simulink model "GSAutopilot"  (R2022b)
settings: Solver=ode45  StartTime=0.0  StopTime=50  RelTol=1e-3  AbsTol=1e-6
PreLoadFcn:
  | x_ini = 0;
  | h_ini = 10000/3.28084;  % 10,000 ft
  | alpha_ini = 0;
  | theta_ini = 0;
  | v_ini = 700;   % m/s
  | q_ini = 0;
model workspace (MATLAB code in the model file):
  | AirframeData
  | Kp0 = 0.1*ones(11,8);
  | Ki0 = 2*ones(11,8);
  | Ka0 = 0.001*ones(11,8);
  | Kg0 = -1000*ones(11,8);
values from neighbouring files (symbols this model uses):
  Cm_alpha = am*al.^3 + bm*al.*abs(al) - cm*(7-8*M/3).*al    [AirframeData.m]
  Cm_el = -0.206000/d2r    (= -11.8029305797)    [AirframeData.m]
  Cm_q = -1.719    [AirframeData.m]
  Cx_alpha = -0.3*ones(length(alpha_vec),length(Mach_vec))    [AirframeData.m]
  Cz_alpha = an*al.^3 + bn*al.*abs(al) + cn*(2-M/3).*al    [AirframeData.m]
  Cz_el = -0.034000/d2r    (= -1.94805650344)    [AirframeData.m]
  d2r = pi/180    (= 0.0174532925199)    [AirframeData.m]
  d_ref = 0.75/m2ft    (= 0.228599992685)    [AirframeData.m]
  fin_max = 30.0*d2r    (= 0.523598775598)    [AirframeData.m]
  fin_min = -30.0*d2r    (= -0.523598775598)    [AirframeData.m]
  g = 9.81    [AirframeData.m]
  S_ref = 0.44/m2ft^2    (= 0.0408773349839)    [AirframeData.m]
  Thrust = 10e3    (= 10000)    [AirframeData.m]
libraries: aerospace x2, simulink x1
settings Model: Creator=The MathWorks, Inc.  LastModifiedBy=cosorio
settings SolverCC: AutoScaleAbsTol=off  AlgebraicLoopSolver=TrustRegion
settings DataIOCC: SaveFormat=Array  ReturnWorkspaceOutputs=off  SignalLoggingName=sigsOut
settings OptimizationCC: BlockReduction=off  BooleanDataType=off  ExpressionDepthLimit=2147483647  InitFltsAndDblsToZero=on  LifeSpan=inf
settings DebuggingCC: SaveWithParameterizedLinksMsg=none  UnderspecifiedInitializationDetection=Classic  MergeDetectMultiDrivingBlocksExec=none  CheckExecutionContextPreStartOutputMsg=on  SignalResolutionControl=TryResolveAllWithWarning  MultiTaskDSMMsg=warning  FcnCallInpInsideContextMsg=warning  UnconnectedInputMsg=warning  UnconnectedOutputMsg=warning  UnconnectedLineMsg=warning  AllowSymbolicDim=off  StateNameClashWarn=warning  SFUnexpectedBacktrackingDiag=warning  SFNoUnconditionalDefaultTransitionDiag=warning  SFExecutionAtInitializationDiag=none  SFMachineParentedDataDiag=warning  ArithmeticOperatorsInVariantConditions=warning
settings HardwareCC: ProdBitPerPointer=32  ProdBitPerSizeT=32  ProdBitPerPtrDiffT=32  ProdLargestAtomicFloat=None  ProdIntDivRoundTo=Undefined  ProdEndianess=Unspecified  ProdWordSize=32  ProdHWDeviceType=32-bit Generic  TargetUnknown=on
settings ModelReferenceCC: EnableRefExpFcnMdlSchedulingChecks=on  PropagateSignalLabelsOutOfModel=off
settings SFSimCC: SimUseLocalCustomCode=off  CustomCodeUndefinedFunction=UseInterfaceOnly
settings RTWCC: RTWUseLocalCustomCode=off
settings CodeAppCC: StateflowObjectComments=on
settings GRTTargetCC: TargetFcnLib=ansi_tfl_tmw.mat  TargetLangStandard=C89/C90 (ANSI)  CombineOutputUpdateFcns=off  GRTInterface=on
settings ConfigComp: CovMetricSettings=dw  CovSaveCumulativeToWorkspaceVar=on  CovSaveSingleToWorkspaceVar=on  CovExternalEMLEnable=off

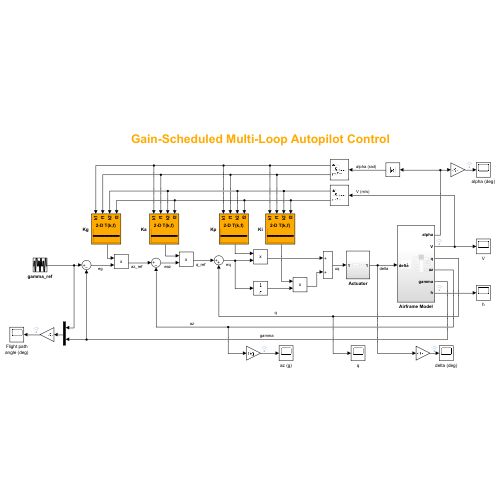
[thumbnail: Simulink's stored preview of the top-level diagram]
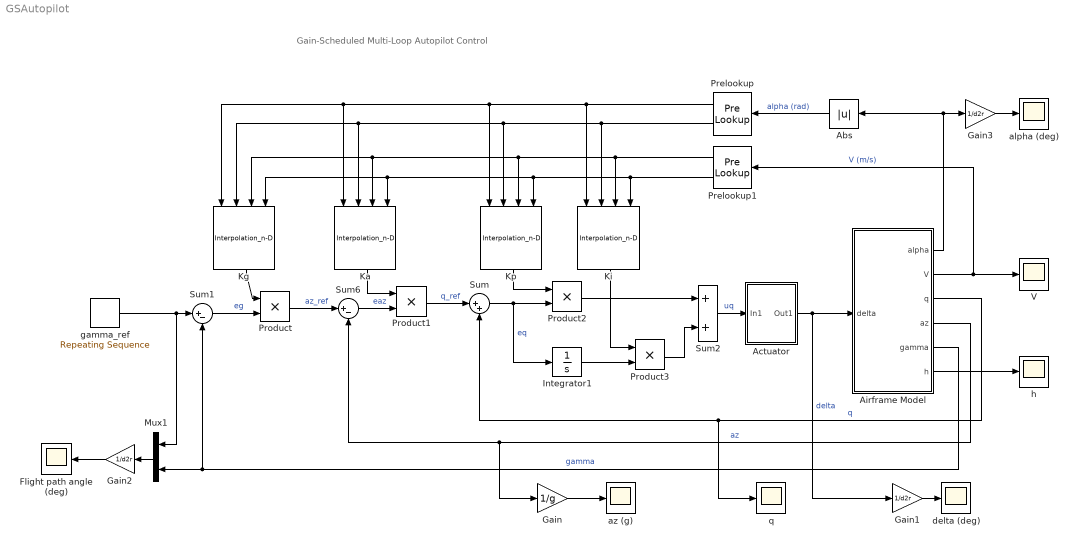
== system GSAutopilot ==
  note: Gain-Scheduled Multi-Loop Autopilot Control
  Abs : Abs  SaturateOnIntegerOverflow=off
  Actuator : Subsystem
  Airframe Model : Subsystem
  Flight path angle (deg) : Scope
  Gain : Gain  Gain=1/g
  Gain1 : Gain  Gain=1/d2r
  Gain2 : Gain  Gain=1/d2r
  Gain3 : Gain  Gain=1/d2r
  Integrator1 : Integrator
  Ka : Interpolation_n-D  Table=Ka0  InternalRulePriority=Speed
  Kg : Interpolation_n-D  Table=Kg0  InternalRulePriority=Speed
  Ki : Interpolation_n-D  Table=Ki0  InternalRulePriority=Speed
  Kp : Interpolation_n-D  Table=Kp0  InternalRulePriority=Speed
  Mux1 : Mux  Inputs=2
  Prelookup : PreLookup  BreakpointsData=(0:2:20)*(pi/180)  ExtrapMethod=Linear
  Prelookup1 : PreLookup  BreakpointsData=700:100:1400  ExtrapMethod=Linear
  Product{,1..3} (4 alike) : Product
  Sum : Sum  Inputs=|++  SaturateOnIntegerOverflow=on
  Sum1 : Sum  Inputs=|+-  SaturateOnIntegerOverflow=on
  Sum2 : Sum  SaturateOnIntegerOverflow=on
  Sum6 : Sum  Inputs=|+-  SaturateOnIntegerOverflow=on
  V : Scope
  alpha (deg) : Scope
  az (g) : Scope
  delta (deg) : Scope
  gamma_ref : simulink/Sources/Repeating Sequence  rep_seq_t=[0 6 8 16 20 26 32 40 44 50]  rep_seq_y=[0 0 pi/6 pi/6 -pi/6 -pi/6 pi/4 pi/4 0 0]
  h : Scope
  q : Scope
  wires:
  Sum/1 -> Product2/2, Integrator1/1  "eq"
  Product3/1 -> Sum2/2
  Airframe Model/4(az) -> Gain/1, Sum6/2  "az"
  Airframe Model/1(alpha) -> Abs/1, Gain3/1
  Product2/1 -> Sum2/1
  Product1/1 -> Sum/1  "q_ref"
  Sum6/1 -> Product1/2  "eaz"
  Actuator/1(Out1) -> Airframe Model/1(delta), Gain1/1  "delta"
  Product/1 -> Sum6/1  "az_ref"
  Sum1/1 -> Product/2  "eg"
  Airframe Model/5(gamma) -> Mux1/2, Sum1/2  "gamma"
  Sum2/1 -> Actuator/1(In1)  "uq"
  Airframe Model/3(q) -> q/1, Sum/2  "q"
  gamma_ref/1 -> Sum1/1, Mux1/1
  Gain/1 -> az (g)/1
  Gain1/1 -> delta (deg)/1
  Mux1/1 -> Gain2/1
  Gain2/1 -> Flight path angle (deg)/1
  Gain3/1 -> alpha (deg)/1
  Airframe Model/2(V) -> Prelookup1/1, V/1  "V (m/s)"
  Airframe Model/6(h) -> h/1
  Kg/1 -> Product/1
  Ka/1 -> Product1/1
  Integrator1/1 -> Product3/2
  Kp/1 -> Product2/1
  Ki/1 -> Product3/1
  Abs/1 -> Prelookup/1  "alpha (rad)"
  Prelookup/1 -> Ka/1, Kg/1, Kp/1, Ki/1
  Prelookup/2 -> Ki/2, Kp/2, Ka/2, Kg/2
  Prelookup1/1 -> Kp/3, Kg/3, Ka/3, Ki/3
  Prelookup1/2 -> Ki/4, Kg/4, Ka/4, Kp/4

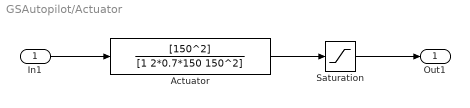
== system GSAutopilot/Actuator ==
  In1 : Inport
  Actuator : TransferFcn  Numerator=[150^2]  Denominator=[1 2*0.7*150 150^2]
  Saturation : Saturate  UpperLimit=fin_max  LowerLimit=fin_min
  Out1 : Outport  VectorParamsAs1DForOutWhenUnconnected=off
  wires:
  Actuator/1 -> Saturation/1
  In1/1 -> Actuator/1
  Saturation/1 -> Out1/1

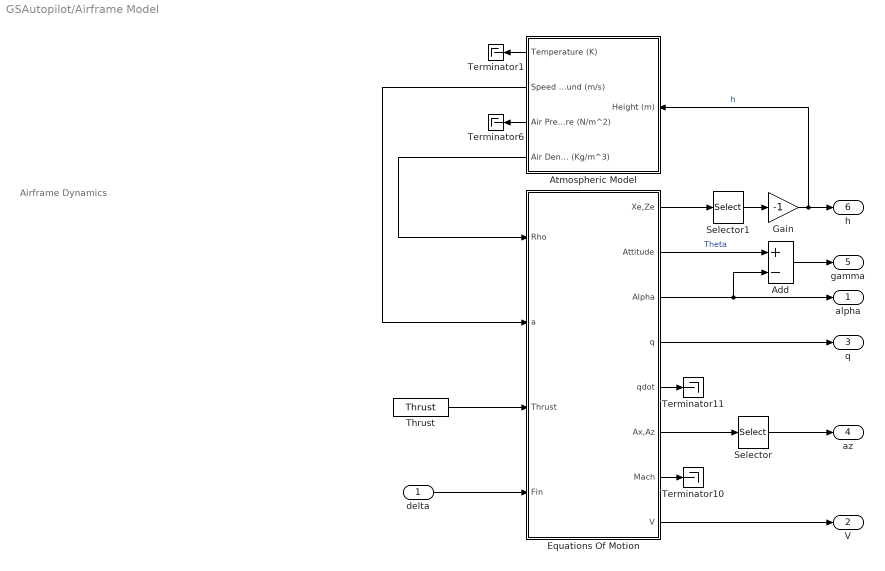
== system GSAutopilot/Airframe Model ==
  note: Airframe Dynamics
  delta : Inport
  Add : Sum  Inputs=+-
  Atmospheric Model : Subsystem  mask(Atmosphere Model){}
      mask help: Compute International Standard Atmosphere (ISA) model for altitudes between 0 Km and 20 Km.
      mask init:
      | g=9.80665; % m/s
      | gamma = 1.4;
      | R = 287.0531; %J/Kg/K
      | L = 0.0065; % K/m
      | h_trop = 11000; % m
      | rho0 = 1.225; %Kg/m^3
      | P0 = 101325; % Pa
      | T0 = 288.15; % K
      mask Help:
      | <p>This block contains the International Standard Atmosphere (ISA) model for altitudes between 0 and 20 Km.  If the height input is greater than 20 Km, the height will be limited to 20 Km.</p>
      | 
      | <p><H4>Block Input</H4>
      | <ul>
      |     <li>Height - Altitude in meters</li>
      | </ul>
      | </p>
      | <p><H4>Block Outputs</H4>
      | <ul>
      |     <li>Temperature - in degree Kelvin</li>
      |     <li>Speed of Sound - in meters/second</li>
      |     <li>Air Pressure - in Pascals</li>
      |     <li>Air Density - in kilograms/meter</li>
      | </ul>
      | </p>
  Equations Of Motion : Subsystem
  Gain : Gain  Gain=-1
  Selector : Selector  InputPortWidth=2  IndexOptions=Index vector (dialog)  Indices=[2]  OutputSizes=1
  Selector1 : Selector  InputPortWidth=2  IndexOptions=Index vector (dialog)  Indices=[2]  OutputSizes=1
  Terminator{1,6,10..11} (4 alike) : Terminator
  Thrust : Constant  Value=Thrust
  alpha : Outport  InitialOutput=0  VectorParamsAs1DForOutWhenUnconnected=off
  V : Outport  Port=2  InitialOutput=0  VectorParamsAs1DForOutWhenUnconnected=off
  q : Outport  Port=3  InitialOutput=0  VectorParamsAs1DForOutWhenUnconnected=off
  az : Outport  Port=4  InitialOutput=0  VectorParamsAs1DForOutWhenUnconnected=off
  gamma : Outport  Port=5  InitialOutput=0  VectorParamsAs1DForOutWhenUnconnected=off
  h : Outport  Port=6  InitialOutput=0  VectorParamsAs1DForOutWhenUnconnected=off
  wires:
  Atmospheric Model/1(Temperature (K)) -> Terminator1/1
  Atmospheric Model/3("Air Pressure (N/m^2) ") -> Terminator6/1
  delta/1 -> Equations Of Motion/4(Fin)
  Equations Of Motion/8(V) -> V/1
  Selector/1 -> az/1
  Atmospheric Model/2("Speed of Sound (m/s) ") -> Equations Of Motion/2(a)
  Atmospheric Model/4(Air Density (Kg/m^3)) -> Equations Of Motion/1(Rho)
  Equations Of Motion/7(Mach) -> Terminator10/1
  Equations Of Motion/5(qdot) -> Terminator11/1
  Equations Of Motion/4(q) -> q/1
  Thrust/1 -> Equations Of Motion/3(Thrust)
  Equations Of Motion/3(Alpha) -> alpha/1, Add/2
  Equations Of Motion/6(Ax,Az) -> Selector/1
  Equations Of Motion/2(Attitude) -> Add/1  "Theta"
  Add/1 -> gamma/1
  Equations Of Motion/1(Xe,Ze) -> Selector1/1
  Selector1/1 -> Gain/1
  Gain/1 -> Atmospheric Model/1(Height (m)), h/1  "h"

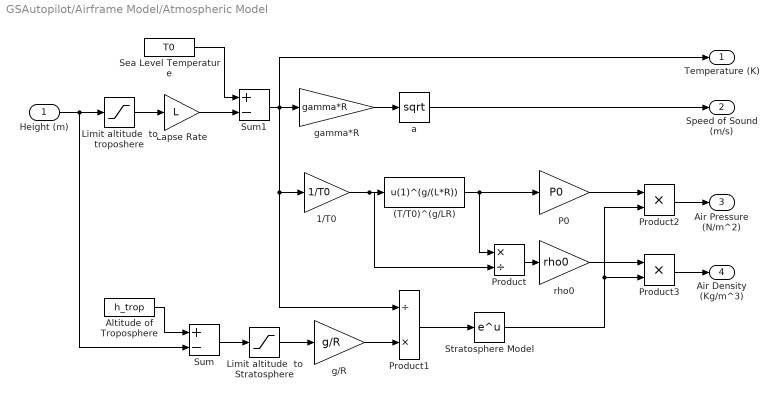
== system GSAutopilot/Airframe Model/Atmospheric Model ==
  Height (m) : Inport
  (T/T0)^(g/LR) : Fcn  Expr=u(1)^(g/(L*R))
  1/T0 : Gain  Gain=1/T0  SaturateOnIntegerOverflow=on  OutDataTypeStr=Inherit: Same as input  ParamDataTypeStr=Inherit: Same as input
  Altitude of Troposphere : Constant  Value=h_trop
  Lapse Rate : Gain  Gain=L  SaturateOnIntegerOverflow=on  OutDataTypeStr=Inherit: Same as input  ParamDataTypeStr=Inherit: Same as input
  Limit altitude  to Stratosphere : Saturate  UpperLimit=0  LowerLimit=h_trop-20000
  Limit altitude  to troposhere : Saturate  UpperLimit=h_trop  LowerLimit=0
  P0 : Gain  Gain=P0  SaturateOnIntegerOverflow=on  OutDataTypeStr=Inherit: Same as input  ParamDataTypeStr=Inherit: Same as input
  Product : Product  Inputs=*/  InputSameDT=on  RndMeth=Zero  SaturateOnIntegerOverflow=on  OutDataTypeStr=Inherit: Same as first input
  Product1 : Product  Inputs=/*  InputSameDT=on  RndMeth=Zero  SaturateOnIntegerOverflow=on  OutDataTypeStr=Inherit: Same as first input
  Product2 : Product  InputSameDT=on  RndMeth=Zero  SaturateOnIntegerOverflow=on  OutDataTypeStr=Inherit: Same as first input
  Product3 : Product  InputSameDT=on  RndMeth=Zero  SaturateOnIntegerOverflow=on  OutDataTypeStr=Inherit: Same as first input
  Sea Level Temperature : Constant  Value=T0
  Stratosphere Model : Math  SignedPower=on
  Sum : Sum  Inputs=+-  InputSameDT=on  SaturateOnIntegerOverflow=on  OutDataTypeStr=Inherit: Same as first input
  Sum1 : Sum  Inputs=+-  InputSameDT=on  SaturateOnIntegerOverflow=on  OutDataTypeStr=Inherit: Same as first input
  a : Math  Operator=sqrt  SignedPower=on
  g/R : Gain  Gain=g/R  SaturateOnIntegerOverflow=on  OutDataTypeStr=Inherit: Same as input  ParamDataTypeStr=Inherit: Same as input
  gamma*R : Gain  Gain=gamma*R  SaturateOnIntegerOverflow=on  OutDataTypeStr=Inherit: Same as input  ParamDataTypeStr=Inherit: Same as input
  rho0 : Gain  Gain=rho0  SaturateOnIntegerOverflow=on  OutDataTypeStr=Inherit: Same as input  ParamDataTypeStr=Inherit: Same as input
  Temperature (K) : Outport  InitialOutput=0  VectorParamsAs1DForOutWhenUnconnected=off
  "Speed of Sound (m/s) " : Outport  Port=2  InitialOutput=0  VectorParamsAs1DForOutWhenUnconnected=off
  "Air Pressure (N/m^2) " : Outport  Port=3  InitialOutput=0  VectorParamsAs1DForOutWhenUnconnected=off
  Air Density (Kg/m^3) : Outport  Port=4  InitialOutput=0  VectorParamsAs1DForOutWhenUnconnected=off
  wires:
  Limit altitude  to Stratosphere/1 -> g/R/1
  Sum/1 -> Limit altitude  to Stratosphere/1
  Altitude of Troposphere/1 -> Sum/1
  Product1/1 -> Stratosphere Model/1
  g/R/1 -> Product1/2
  Stratosphere Model/1 -> Product3/2, Product2/2
  Product3/1 -> Air Density (Kg/m^3)/1
  rho0/1 -> Product3/1
  Product2/1 -> "Air Pressure (N/m^2) "/1
  P0/1 -> Product2/1
  Sea Level Temperature/1 -> Sum1/1
  Lapse Rate/1 -> Sum1/2
  Sum1/1 -> Product1/1, 1/T0/1, gamma*R/1, Temperature (K)/1
  a/1 -> "Speed of Sound (m/s) "/1
  gamma*R/1 -> a/1
  1/T0/1 -> (T/T0)^(g/LR)/1, Product/2
  (T/T0)^(g/LR)/1 -> P0/1, Product/1
  Product/1 -> rho0/1
  Limit altitude  to troposhere/1 -> Lapse Rate/1
  Height (m)/1 -> Sum/2, Limit altitude  to troposhere/1

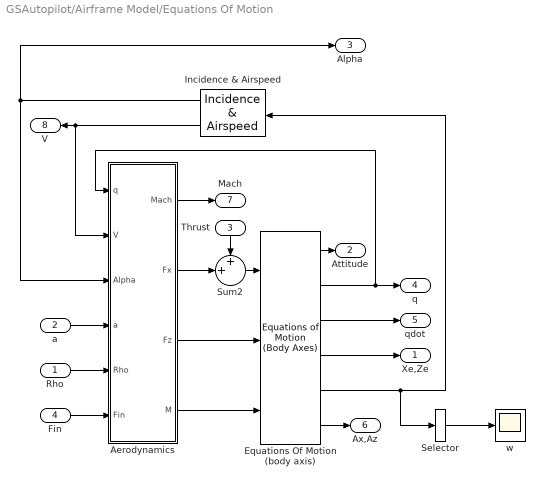
== system GSAutopilot/Airframe Model/Equations Of Motion ==
  Rho : Inport
  a : Inport  Port=2
  Thrust : Inport  Port=3
  Fin : Inport  Port=4
  " Equations Of Motion (body axis)" : aerospace/3DoF Equations of Motion / Equations of Motion (Body Axes)  v_ini=v_ini  theta_ini=theta_ini  alpha_ini=alpha_ini  q_ini=q_ini  pos_ini=[x_ini -h_ini]  mass=mass  Iyy=Iyy  g=g
  Aerodynamics : Subsystem
  Incidence & Airspeed : aerospace/3DoF Equations of Motion /Incidence  & Airspeed
  Selector : Selector  InputPortWidth=2  IndexOptions=Index vector (dialog)  Indices=[2]  OutputSizes=1
  Sum2 : Sum  Inputs=++|  InputSameDT=on  SaturateOnIntegerOverflow=on  OutDataTypeStr=Inherit: Same as first input
  w : Scope
  Xe,Ze : Outport  InitialOutput=0  VectorParamsAs1DForOutWhenUnconnected=off
  Attitude : Outport  Port=2  InitialOutput=0  VectorParamsAs1DForOutWhenUnconnected=off
  Alpha : Outport  Port=3  InitialOutput=0  VectorParamsAs1DForOutWhenUnconnected=off
  q : Outport  Port=4  InitialOutput=0  VectorParamsAs1DForOutWhenUnconnected=off
  qdot : Outport  Port=5  InitialOutput=0  VectorParamsAs1DForOutWhenUnconnected=off
  Ax,Az : Outport  Port=6  InitialOutput=0  VectorParamsAs1DForOutWhenUnconnected=off
  Mach : Outport  Port=7  InitialOutput=0  VectorParamsAs1DForOutWhenUnconnected=off
  V : Outport  Port=8  InitialOutput=0  VectorParamsAs1DForOutWhenUnconnected=off
  wires:
  " Equations Of Motion (body axis)"/5 -> Selector/1, Incidence & Airspeed/1
  " Equations Of Motion (body axis)"/6 -> Ax,Az/1
  " Equations Of Motion (body axis)"/4 -> Xe,Ze/1
  " Equations Of Motion (body axis)"/1 -> Attitude/1
  " Equations Of Motion (body axis)"/3 -> qdot/1
  " Equations Of Motion (body axis)"/2 -> Aerodynamics/1(q), q/1
  Thrust/1 -> Sum2/1
  Aerodynamics/2(Fx) -> Sum2/2
  Aerodynamics/3(Fz) -> " Equations Of Motion (body axis)"/2
  Incidence & Airspeed/2 -> Aerodynamics/2(V), V/1
  Fin/1 -> Aerodynamics/6(Fin)
  a/1 -> Aerodynamics/4(a)
  Rho/1 -> Aerodynamics/5(Rho)
  Incidence & Airspeed/1 -> Alpha/1, Aerodynamics/3(Alpha)
  Sum2/1 -> " Equations Of Motion (body axis)"/1
  Aerodynamics/4(" M") -> " Equations Of Motion (body axis)"/3
  Aerodynamics/1(" Mach") -> Mach/1
  Selector/1 -> w/1

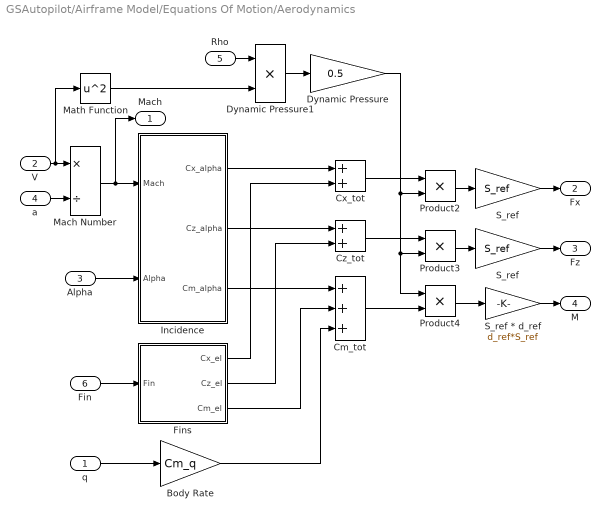
== system GSAutopilot/Airframe Model/Equations Of Motion/Aerodynamics ==
  q : Inport
  V : Inport  Port=2
  Alpha : Inport  Port=3
  a : Inport  Port=4
  Rho : Inport  Port=5
  Fin : Inport  Port=6
  Body Rate : Gain  Gain=Cm_q  SaturateOnIntegerOverflow=on  OutDataTypeStr=Inherit: Same as input  ParamDataTypeStr=Inherit: Same as input
  Cm_tot : Sum  Inputs=+++  InputSameDT=on  SaturateOnIntegerOverflow=on  OutDataTypeStr=Inherit: Same as first input
  Cx_tot : Sum  InputSameDT=on  SaturateOnIntegerOverflow=on  OutDataTypeStr=Inherit: Same as first input
  Cz_tot : Sum  InputSameDT=on  SaturateOnIntegerOverflow=on  OutDataTypeStr=Inherit: Same as first input
  Dynamic Pressure : Gain  Gain=0.5  SaturateOnIntegerOverflow=on  OutDataTypeStr=Inherit: Same as input  ParamDataTypeStr=Inherit: Same as input
  Dynamic Pressure1 : Product  InputSameDT=on  SaturateOnIntegerOverflow=on  OutDataTypeStr=Inherit: Same as first input
  Fins : Subsystem
  Incidence : Subsystem
  Mach Number : Product  Inputs=*/  InputSameDT=on  SaturateOnIntegerOverflow=on  OutDataTypeStr=Inherit: Same as first input
  Math Function : Math  Operator=square  SignedPower=on
  Product2 : Product  InputSameDT=on  SaturateOnIntegerOverflow=on  OutDataTypeStr=Inherit: Same as first input
  Product3 : Product  InputSameDT=on  SaturateOnIntegerOverflow=on  OutDataTypeStr=Inherit: Same as first input
  Product4 : Product  InputSameDT=on  SaturateOnIntegerOverflow=on  OutDataTypeStr=Inherit: Same as first input
  S_ref : Gain  Gain=S_ref  SaturateOnIntegerOverflow=on  OutDataTypeStr=Inherit: Same as input  ParamDataTypeStr=Inherit: Same as input
  S_ref * d_ref : Gain  Gain=d_ref*S_ref  SaturateOnIntegerOverflow=on  OutDataTypeStr=Inherit: Same as input  ParamDataTypeStr=Inherit: Same as input
  "S_ref " : Gain  Gain=S_ref  SaturateOnIntegerOverflow=on  OutDataTypeStr=Inherit: Same as input  ParamDataTypeStr=Inherit: Same as input
  " Mach" : Outport  InitialOutput=0  VectorParamsAs1DForOutWhenUnconnected=off
  Fx : Outport  Port=2  InitialOutput=[0]  VectorParamsAs1DForOutWhenUnconnected=off
  Fz : Outport  Port=3  InitialOutput=0  VectorParamsAs1DForOutWhenUnconnected=off
  " M" : Outport  Port=4  InitialOutput=0  VectorParamsAs1DForOutWhenUnconnected=off
  wires:
  Mach Number/1 -> Incidence/1(Mach), " Mach"/1
  q/1 -> Body Rate/1
  Cm_tot/1 -> Product4/2
  Product4/1 -> S_ref * d_ref/1
  S_ref * d_ref/1 -> " M"/1
  Fin/1 -> Fins/1(Fin)
  "S_ref "/1 -> Fz/1
  Product3/1 -> "S_ref "/1
  S_ref/1 -> Fx/1
  Product2/1 -> S_ref/1
  Cz_tot/1 -> Product3/1
  Cx_tot/1 -> Product2/1
  Alpha/1 -> Incidence/2(Alpha)
  a/1 -> Mach Number/2
  Body Rate/1 -> Cm_tot/3
  Fins/3(Cm_el) -> Cm_tot/2
  Incidence/3(Cm_alpha) -> Cm_tot/1
  Fins/2(Cz_el) -> Cz_tot/2
  Incidence/2(Cz_alpha) -> Cz_tot/1
  Fins/1(Cx_el) -> Cx_tot/2
  Incidence/1(Cx_alpha) -> Cx_tot/1
  V/1 -> Mach Number/1, Math Function/1
  Dynamic Pressure/1 -> Product4/1, Product3/2, Product2/2
  Dynamic Pressure1/1 -> Dynamic Pressure/1
  Rho/1 -> Dynamic Pressure1/1
  Math Function/1 -> Dynamic Pressure1/2

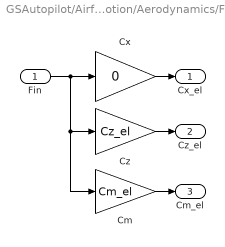
== system GSAutopilot/Airframe Model/Equations Of Motion/Aerodynamics/Fins ==
  Fin : Inport
  Cm : Gain  Gain=Cm_el  SaturateOnIntegerOverflow=on  OutDataTypeStr=Inherit: Same as input  ParamDataTypeStr=Inherit: Same as input
  Cx : Gain  Gain=0  SaturateOnIntegerOverflow=on  OutDataTypeStr=Inherit: Same as input  ParamDataTypeStr=Inherit: Same as input
  Cz : Gain  Gain=Cz_el  SaturateOnIntegerOverflow=on  OutDataTypeStr=Inherit: Same as input  ParamDataTypeStr=Inherit: Same as input
  Cx_el : Outport  InitialOutput=0  VectorParamsAs1DForOutWhenUnconnected=off
  Cz_el : Outport  Port=2  InitialOutput=0  VectorParamsAs1DForOutWhenUnconnected=off
  Cm_el : Outport  Port=3  InitialOutput=0  VectorParamsAs1DForOutWhenUnconnected=off
  wires:
  Cz/1 -> Cz_el/1
  Cm/1 -> Cm_el/1
  Cx/1 -> Cx_el/1
  Fin/1 -> Cz/1, Cm/1, Cx/1

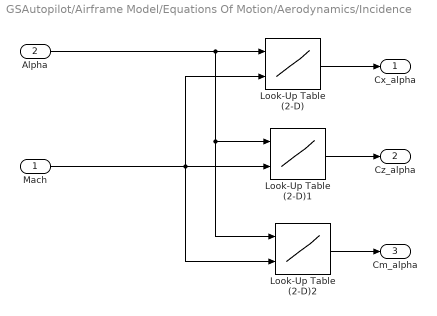
== system GSAutopilot/Airframe Model/Equations Of Motion/Aerodynamics/Incidence ==
  Mach : Inport
  Alpha : Inport  Port=2
  Look-Up Table (2-D) : Lookup2D  RowIndex=alpha_vec  ColumnIndex=Mach_vec  Table=Cx_alpha  InputSameDT=off
  Look-Up Table (2-D)1 : Lookup2D  RowIndex=alpha_vec  ColumnIndex=Mach_vec  Table=Cz_alpha  InputSameDT=off
  Look-Up Table (2-D)2 : Lookup2D  RowIndex=alpha_vec  ColumnIndex=Mach_vec  Table=Cm_alpha  InputSameDT=off
  Cx_alpha : Outport  InitialOutput=0  VectorParamsAs1DForOutWhenUnconnected=off
  Cz_alpha : Outport  Port=2  InitialOutput=0  VectorParamsAs1DForOutWhenUnconnected=off
  Cm_alpha : Outport  Port=3  InitialOutput=0  VectorParamsAs1DForOutWhenUnconnected=off
  wires:
  Mach/1 -> Look-Up Table (2-D)2/2, Look-Up Table (2-D)1/2, Look-Up Table (2-D)/2
  Alpha/1 -> Look-Up Table (2-D)2/1, Look-Up Table (2-D)1/1, Look-Up Table (2-D)/1
  Look-Up Table (2-D)2/1 -> Cm_alpha/1
  Look-Up Table (2-D)1/1 -> Cz_alpha/1
  Look-Up Table (2-D)/1 -> Cx_alpha/1
